simulink model "CrashAlgo_TestEnvironment_MotorradJan"  (R2019a)
settings: Solver=FixedStepAuto  StartTime=0.0  StopTime=data.timeVectorAcc(end)  FixedStep=0.01  RelTol=1e-3
undefined symbols (not defined in the file or in its folder): data, timeVector
libraries: simulink x1
settings Model: Creator=snj7rt  LastModifiedBy=snj7rt
settings DataIOCC: ReturnWorkspaceOutputs=off
settings DebuggingCC: ArithmeticOperatorsInVariantConditions=warning
settings SFSimCC: SimUseLocalCustomCode=off
settings RTWCC: RTWUseLocalCustomCode=off
settings CodeAppCC: StateflowObjectComments=on

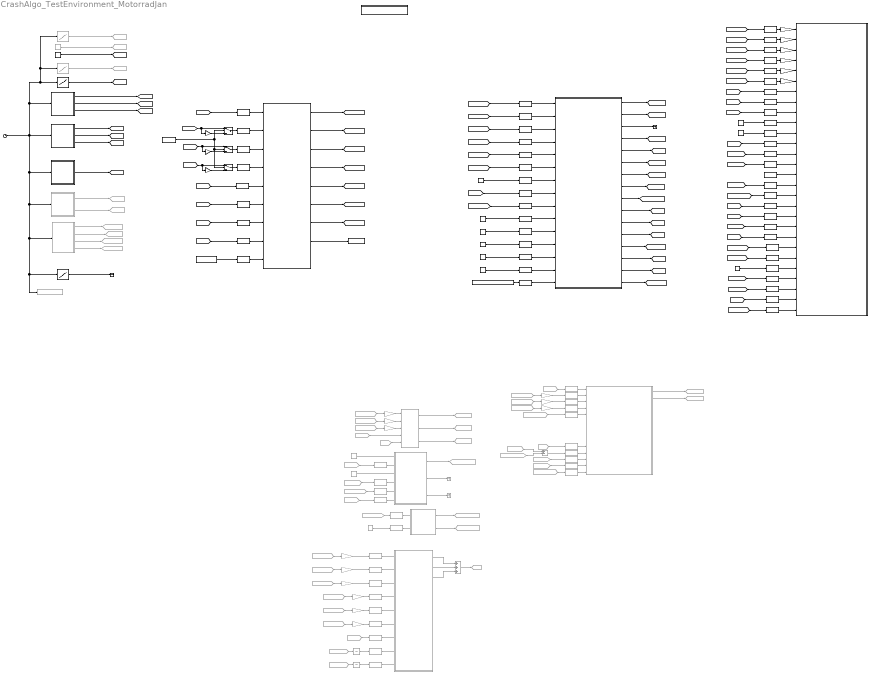
== system CrashAlgo_TestEnvironment_MotorradJan ==
  note: TestSetup for kalman extension regarding longitudinal acceleration compensation
  Acc_X1 : Lookup_n-D  Commented=on  NumberOfTableDimensions=1  BreakpointsForDimension1=timeVector(1:length([ones(floor(0.3*length(timeVector)),1);zeros(floor(0.7*length(timeVector)),1)]))  BreakpointsForDimension3=[5, 7]  Table=[20*ones(floor(0.3*length(timeVector)),1);zeros(floor(0.7*length(timeVector)),1)]  InternalRulePriority=Speed  RndMeth=Simplest  InputSameDT=on
  Accelerometer : Subsystem
  Add : Sum  Commented=on  Inputs=+-
  Add1 : Sum  Commented=on  Inputs=+++
  Barometer : Subsystem
  Chart1 : Stateflow chart  Commented=on  BlockKeywords=__PRM__SERIALIZED__DATA__:Stateflow Chart,Stateflow Diagram  TreatAsAtomicUnit=on
  Clock : Clock
  Constant : Constant  Value=data.osType
  Constant{1,3,8,11..12} (5 alike) : Constant  Value=0
  Constant10 : Constant  Value=data.InitRotMatFromLogFile
  Constant13 : Constant  Value=data.longAccCompForEulerEstFlagFromWorkspace
  Constant2 : Constant  Commented=on  Value=20
  Constant4 : Constant
  Constant46 : Constant  Commented=on  Value=10
  Constant47 : Constant  Commented=on  Value=0.1
  Constant5 : Constant  Value=2
  Constant6 : Constant  Value=5
  Constant7 : Constant  Value=7
  Constant9 : Constant  Commented=on  Value=2
  Data Type Conversion{,41,51..53,55..57,59..70,73,75} (22 alike) : DataTypeConversion  Commented=on  OutDataTypeStr=single
  Data Type Conversion{1..20,22..26,42..43,58} (28 alike) : DataTypeConversion
  Data Type Conversion{21,27..40,44..50,54,76} (24 alike) : DataTypeConversion  RndMeth=Zero
  Data Type Conversion71 : DataTypeConversion  Commented=on  OutDataTypeStr=int16
  Data Type Conversion72 : DataTypeConversion  Commented=on  OutDataTypeStr=int16
  Data Type Conversion74 : DataTypeConversion  Commented=on  OutDataTypeStr=int16
  Double-Click Button to set current folder : Subsystem
      settings: OpenFcn=cd(fileparts(get_param(gcs,'filename')));
      mask Display: disp('\bf\fontsize{16}Double-Click to set current folder      ','texmode','on')
  DuAcc : Subsystem  Commented=on
  FilterButterworth : Subsystem  Commented=on
  From{6,14,31,71} (4 alike) : From  Commented=on  GotoTag=StepTime
  From15 : From  Commented=on  GotoTag=accBfFiltX_g
  From18 : From  Commented=on  GotoTag=accBfFiltY_g
  From19 : From  Commented=on  GotoTag=accBfFiltZ_g
  From20 : From  Commented=on  GotoTag=accBf_X_mg
  From21 : From  Commented=on  GotoTag=accBf_Y_mg
  From22 : From  Commented=on  GotoTag=accBf_Z_mg
  From23 : From  Commented=on  GotoTag=accBfFiltX_g
  From30 : From  Commented=on  GotoTag=calibFlag
  From32 : From  Commented=on  GotoTag=reinitializeEulerEstimation
  From33 : From  Commented=on  GotoTag=SecondCalibrationDelayed
  From34 : From  Commented=on  GotoTag=gyrBf_X_mdegs
  From35 : From  Commented=on  GotoTag=gyrBf_Y_mdegs
  From36 : From  Commented=on  GotoTag=gyrBf_Z_mdegs
  From37 : From  Commented=on  GotoTag=gyrBf_X_mdegs
  From38 : From  Commented=on  GotoTag=eulerPitchComp_deg
  From39 : From  Commented=on  GotoTag=accBf_X_mg
  From40 : From  Commented=on  GotoTag=accBf_Y_mg
  From41 : From  Commented=on  GotoTag=accBf_Z_mg
  From42 : From  Commented=on  GotoTag=varSum
  From43 : From  Commented=on  GotoTag=varSum
  From44 : From  Commented=on  GotoTag=gyrBf_Y_mdegs
  From45 : From  Commented=on  GotoTag=gyrBf_Z_mdegs
  From47 : From  Commented=on  GotoTag=calibFlag
  From5 : From  Commented=on  GotoTag=Du_Speed
  From7 : From  Commented=on  GotoTag=longAccSpeedBased_g
  From95 : From  Commented=on  GotoTag=eulerRollComp_deg
  Gain{,1..5} (6 alike) : Gain  Gain=1/1000
  Gain{9..20} (12 alike) : Gain  Commented=on  Gain=1/1000
  Gain6 : Gain  Gain=-1
  Gain7 : Gain  Gain=-1
  Gain8 : Gain  Gain=-1
  Goto153 : Goto  Commented=on  GotoTag=longAccSpeedBased_g
  Goto16 : Goto  Commented=on  GotoTag=Du_Cadence
  Goto19 : Goto  Commented=on  GotoTag=Du_Speed
  Goto20 : Goto  Commented=on  GotoTag=initMountingAngleDeg
  Goto21 : Goto  Commented=on  GotoTag=accBfFiltX_g
  Goto22 : Goto  Commented=on  GotoTag=initMountingSetup
  Goto24 : Goto  Commented=on  GotoTag=DuAccX_mg
  Goto25 : Goto  Commented=on  GotoTag=DuAccZ_mg
  Goto26 : Goto  Commented=on  GotoTag=cobiHubConnection
  Goto27 : Goto  Commented=on  GotoTag=hubSetup
  Goto28 : Goto  Commented=on  GotoTag=accBfFiltY_g
  Goto29 : Goto  Commented=on  GotoTag=accBfFiltZ_g
  Goto3 : Goto  Commented=on  GotoTag=Du_Speed
  Goto30 : Goto  Commented=on  GotoTag=SecondCalibrationDelayed
  Goto31 : Goto  Commented=on  GotoTag=eulerRollComp_deg
  Goto32 : Goto  Commented=on  GotoTag=eulerPitchComp_deg
  Goto38 : Goto  Commented=on  GotoTag=varSum
  Goto57 : Goto  Commented=on  GotoTag=reinitializeEulerEstimation
  Gyroscope : Subsystem
  MATLAB Function : MATLAB Function  Commented=on  TreatAsAtomicUnit=on
  MATLAB Function2 : MATLAB Function  Commented=on  TreatAsAtomicUnit=on
  Model : ModelReference  ModelNameDialog=CalibrationMotorbike.slx  SimulationMode=Normal  ModelReferenceVersion=1.1438
  Model2 : ModelReference  ModelNameDialog=CRCL.slx  SimulationMode=Normal  ModelReferenceVersion=1.1949
  Model3 : ModelReference  ModelNameDialog=CrashAlgoSchnee_v2_analysis.slx  SimulationMode=Normal  ModelReferenceVersion=1.56
  SampleTime1 : Constant  Value=0.01
  Switch : Switch  Threshold=2
  Switch1 : Switch  Threshold=2
  Switch2 : Switch  Threshold=2
  Terminator : Terminator
  Terminator1 : Terminator
  Terminator2 : Terminator  Commented=on
  Terminator3 : Terminator  Commented=on
  To Workspace : ToWorkspace  VariableName=estRotMat  SampleTime=-1
  To Workspace2 : ToWorkspace  Commented=on  VariableName=simTimeVector  SampleTime=-1
      settings: Save2DSignal=2-D array (concatenate along first dimension)
  Unit Delay4 : UnitDelay  Commented=on  SampleTime=-1  HasFrameUpgradeWarning=on
  Unit Delay5 : UnitDelay  Commented=on  SampleTime=-1  HasFrameUpgradeWarning=on
  cadence : Lookup_n-D  Commented=on  NumberOfTableDimensions=1  BreakpointsForDimension1=data.timeVectorAcc  BreakpointsForDimension3=[5, 7]  Table=data.cadence_rpm  InternalRulePriority=Speed  RndMeth=Simplest  InputSameDT=on
  cobiSignals : Subsystem  Commented=on
  detectedCrashClass : Lookup_n-D  NumberOfTableDimensions=1  BreakpointsForDimension1=data.timeVectorAcc  BreakpointsForDimension3=[5, 7]  Table=data.crashClass  InternalRulePriority=Speed  RndMeth=Simplest  InputSameDT=on
  risingEdgeTrigger_RET : Stateflow chart  Commented=on  TreatAsAtomicUnit=on
  speed : Lookup_n-D  NumberOfTableDimensions=1  BreakpointsForDimension1=data.timeVectorAcc  BreakpointsForDimension3=[5, 7]  Table=data.speed_kmh  InternalRulePriority=Speed  RndMeth=Simplest  InputSameDT=on
  wires:
  Accelerometer/1(accSfX [mg]) -> [accSfX_mg]  "accSfXEnv_mg"
  Accelerometer/2(accSfY [mg]) -> [accSfY_mg]  "accSfYEnv_mg"
  Accelerometer/3(accSfZ [mg]) -> [accSfZ_mg]  "accSfZEnv_mg"
  Clock/1 -> cadence/1, Acc_X1/1, speed/1, Accelerometer/1(input_Time), Gyroscope/1(input_Time), DuAcc/1(input_Time), To Workspace2/1, detectedCrashClass/1, cobiSignals/1(In1), Barometer/1(input_Time)
  SampleTime1/1 -> [StepTime]
  Gyroscope/2(gyrSfY [mdeg/s]) -> [gyrSfY_mdegs]  "BMI_GYRO_Y"
  Gyroscope/1(gyrSfX [mdeg/s]) -> [gyrSfX_mdegs]  "BMI_GYRO_X"
  Gyroscope/3(gyrSfZ [mdeg/s]) -> [gyrSfZ_mdegs]  "BMI_GYRO_Z"
  Barometer/1(BME_pressure) -> [BMP_pressure]  "BME_pressure"
  Data Type Conversion14/1 -> Model3/15
  Data Type Conversion3/1 -> Gain1/1
  Data Type Conversion16/1 -> Model3/17
  Data Type Conversion9/1 -> Model3/8
  [eulerPitch_deg] -> Data Type Conversion42/1
  Data Type Conversion31/1 -> Model2/5
  [standFire] -> Data Type Conversion17/1
  Constant12/1 -> Data Type Conversion24/1
  [gyrBf_Y_mdegs] -> Data Type Conversion6/1
  Data Type Conversion19/1 -> Model3/20
  Data Type Conversion36/1 -> Model2/10
  Data Type Conversion29/1 -> Model2/3
  Data Type Conversion8/1 -> Model3/7
  Model2/6 -> [TO_curAngleDeg]
  Data Type Conversion5/1 -> Gain3/1
  Data Type Conversion42/1 -> Model3/9
  [gyrBf_X_mdegs] -> Data Type Conversion5/1
  [secondCalibDelayed] -> Data Type Conversion23/1
  [gyrBf_Z_mdegs] -> Data Type Conversion7/1
  [HD_collisionHitFire] -> Data Type Conversion15/1
  Constant5/1 -> Data Type Conversion36/1
  Data Type Conversion11/1 -> Model3/12
  Data Type Conversion28/1 -> Model2/2
  [calibFlag] -> Data Type Conversion22/1
  Data Type Conversion7/1 -> Gain5/1
  [HD_groundHitFire] -> Data Type Conversion13/1
  Model2/5 -> [TO_fire]
  [crashConfidenceLevel] -> Data Type Conversion26/1
  [Du_Speed] -> Data Type Conversion34/1
  [crashFire] -> Data Type Conversion19/1
  [StepTime] -> Data Type Conversion8/1
  Data Type Conversion32/1 -> Model2/6
  Model2/7 -> [HD_groundHitFire]
  Constant7/1 -> Data Type Conversion43/1
  Data Type Conversion43/1 -> Model3/10
  Data Type Conversion20/1 -> Model3/21
  Data Type Conversion15/1 -> Model3/16
  Constant6/1 -> Data Type Conversion10/1
  Data Type Conversion34/1 -> Model2/8
  Data Type Conversion27/1 -> Model2/1
  Data Type Conversion22/1 -> Model3/22
  Data Type Conversion23/1 -> Model3/23
  [RD_fire] -> Data Type Conversion18/1
  Data Type Conversion30/1 -> Model2/4
  Constant11/1 -> Data Type Conversion33/1
  Data Type Conversion17/1 -> Model3/18
  Data Type Conversion10/1 -> Model3/11
  Data Type Conversion6/1 -> Gain4/1
  [TO_curAngleDeg] -> Data Type Conversion12/1
  Data Type Conversion24/1 -> Model3/24
  Data Type Conversion25/1 -> Model3/25
  [HD_collisionHitCurVarSum] -> Data Type Conversion16/1
  [TO_fire] -> Data Type Conversion11/1
  [accBf_Z_mg] -> Data Type Conversion4/1
  Data Type Conversion2/1 -> Gain/1
  Data Type Conversion18/1 -> Model3/19
  [accBf_X_mg] -> Data Type Conversion2/1
  Model2/4 -> [crashConfidenceLevel]
  Model2/1 -> [crashFire]  "CrashFire"
  Data Type Conversion13/1 -> Model3/14
  Data Type Conversion35/1 -> Model2/9
  [eulerRoll_deg] -> Data Type Conversion9/1
  Data Type Conversion4/1 -> Gain2/1
  [accBf_Y_mg] -> Data Type Conversion3/1
  Data Type Conversion26/1 -> Model3/26
  [calibFlag] -> Data Type Conversion35/1
  [HD_hitDirection] -> Data Type Conversion20/1
  Data Type Conversion33/1 -> Model2/7
  Data Type Conversion12/1 -> Model3/13
  [Du_Speed] -> Data Type Conversion1/1
  Data Type Conversion1/1 -> Model3/27
  [BMP_pressure] -> Data Type Conversion45/1
  Data Type Conversion45/1 -> Model/1
  Data Type Conversion46/1 -> Model/2
  Data Type Conversion47/1 -> Model/3
  Data Type Conversion21/1 -> Model/4
  Data Type Conversion44/1 -> Model/5
  Data Type Conversion48/1 -> Model/6
  Data Type Conversion49/1 -> Model/7
  Data Type Conversion50/1 -> Model/8
  Constant2/1 -> Goto3/1
  Model/1 -> [accBf_X_mg]
  Model/2 -> [accBf_Y_mg]
  Model/3 -> [accBf_Z_mg]
  Model/4 -> [gyrBf_X_mdegs]
  Model/5 -> [gyrBf_Y_mdegs]
  Model/6 -> [gyrBf_Z_mdegs]
  Model/7 -> [calibFlag]
  speed/1 -> [Du_Speed]
  [Du_Speed] -> Data Type Conversion50/1
  Acc_X1/1 -> Goto19/1
  Data Type Conversion40/1 -> Model2/14
  Constant3/1 -> Data Type Conversion40/1
  [accBf_X_mg] -> Data Type Conversion27/1
  [accBf_Y_mg] -> Data Type Conversion28/1
  [accBf_Z_mg] -> Data Type Conversion29/1
  [gyrBf_X_mdegs] -> Data Type Conversion30/1
  [gyrBf_Y_mdegs] -> Data Type Conversion31/1
  [gyrBf_Z_mdegs] -> Data Type Conversion32/1
  [SmartphoneDropOutFire] -> Data Type Conversion58/1
  Data Type Conversion58/1 -> Model3/28
  Model2/2 -> [crashScenario]
  [crashScenario] -> Data Type Conversion25/1
  detectedCrashClass/1 -> Terminator/1  "savedCrashClass"
  cobiSignals/1(cobiHubConnection) -> Goto26/1
  cobiSignals/2(cobiHubSetup) -> Goto27/1
  cobiSignals/3(cobiMountingAngle) -> Goto20/1  "InitMountingAngle"
  cobiSignals/4(cobiMountingSetup) -> Goto22/1
  DuAcc/1(DuAccX  [mg]) -> Goto24/1
  DuAcc/2(DuAccZ [mg]) -> Goto25/1
  Model2/3 -> Terminator1/1
  Model2/16 -> [SmartphoneDropOutFire]
  cadence/1 -> Goto16/1
  Gain/1 -> Model3/1
  Gain1/1 -> Model3/2
  Gain2/1 -> Model3/3
  Gain3/1 -> Model3/4
  Gain4/1 -> Model3/5
  Gain5/1 -> Model3/6
  Constant1/1 -> Data Type Conversion37/1
  Data Type Conversion37/1 -> Model2/11
  Constant4/1 -> Data Type Conversion38/1
  Data Type Conversion38/1 -> Model2/12
  Constant8/1 -> Data Type Conversion39/1
  Data Type Conversion39/1 -> Model2/13
  Data Type Conversion54/1 -> Model/9
  Constant10/1 -> Data Type Conversion54/1
  Model/8 -> To Workspace/1
  Model2/8 -> [HD_collisionHitFire]
  Model2/9 -> [HD_collisionHitCurVarSum]
  Model2/10 -> [standFire]
  Model2/11 -> [RD_fire]
  Model2/12 -> [HD_hitDirection]
  Model2/13 -> [secondCalibDelayed]
  Model2/14 -> [eulerPitch_deg]
  Model2/15 -> [eulerRoll_deg]
  [accSfX_mg] -> Gain6/1, Switch/1
  [accSfY_mg] -> Gain7/1, Switch1/1
  [accSfZ_mg] -> Gain8/1, Switch2/1
  [gyrSfZ_mdegs] -> Data Type Conversion49/1
  [gyrSfY_mdegs] -> Data Type Conversion48/1
  Switch1/1 -> Data Type Conversion47/1
  Switch2/1 -> Data Type Conversion21/1
  [gyrSfX_mdegs] -> Data Type Conversion44/1
  Switch/1 -> Data Type Conversion46/1
  Constant/1 -> Switch2/2, Switch1/2, Switch/2
  Gain6/1 -> Switch/3
  Gain7/1 -> Switch1/3
  Gain8/1 -> Switch2/3
  Constant46/1 -> Chart1/1(LAE_minSpeed_kmh)
  Chart1/1(LAE_longAcc_g) -> Goto153/1  "LAE_longAcc_g"
  Constant47/1 -> Chart1/3(LAE_minSpeedDelta_kmh)
  From5/1 -> Data Type Conversion/1
  MATLAB Function/1(pitch_deg) -> Goto31/1  "pitchKalmanAccComp_deg"
  From6/1 -> Data Type Conversion41/1
  FilterButterworth/3(Z_filt) -> Goto29/1  "accBfFiltZ"
  FilterButterworth/1(X_filt) -> Goto21/1  "accBfFiltX"
  FilterButterworth/2(Y_filt) -> Goto28/1  "accBfFiltY"
  From22/1 -> Gain11/1
  From21/1 -> Gain9/1
  From20/1 -> Gain10/1
  Gain10/1 -> FilterButterworth/1(X)
  Gain9/1 -> FilterButterworth/2(Y)
  Gain11/1 -> FilterButterworth/3(Z)
  From14/1 -> FilterButterworth/4(SampleTime)
  From18/1 -> Data Type Conversion59/1
  From19/1 -> Data Type Conversion60/1
  risingEdgeTrigger_RET/1(RET_output) -> Goto57/1  "reinitEulerEstimation"
  From47/1 -> Data Type Conversion71/1
  risingEdgeTrigger_RET/2(RET_OutDelayed) -> Goto30/1  "secCalibDone Delayed"
  Constant9/1 -> Data Type Conversion72/1  "delayTime"
  From33/1 -> Data Type Conversion61/1
  From32/1 -> Data Type Conversion55/1
  From35/1 -> Gain13/1
  From34/1 -> Gain12/1
  From36/1 -> Gain14/1
  Gain12/1 -> Data Type Conversion51/1
  Gain13/1 -> Data Type Conversion52/1
  Gain14/1 -> Data Type Conversion53/1
  Add/1 -> Data Type Conversion57/1  "accBfXKalmanIn_g"
  From7/1 -> Add/2
  From15/1 -> Add/1
  Gain20/1 -> Data Type Conversion66/1
  Gain17/1 -> Data Type Conversion64/1
  Unit Delay5/1 -> Data Type Conversion70/1
  Gain16/1 -> Data Type Conversion63/1
  Gain18/1 -> Data Type Conversion65/1
  From38/1 -> Unit Delay5/1
  Add1/1 -> Goto38/1  "accVarSum"
  Unit Delay4/1 -> Data Type Conversion69/1
  Gain15/1 -> Data Type Conversion62/1
  From71/1 -> Data Type Conversion68/1
  Gain19/1 -> Data Type Conversion67/1
  MATLAB Function2/1(varAccX) -> Add1/1  "varAccX"
  MATLAB Function2/2(varAccY) -> Add1/2  "varAccY"
  From95/1 -> Unit Delay4/1
  From42/1 -> FilterButterworth/5("accVarSum ")
  From43/1 -> Data Type Conversion56/1
  MATLAB Function2/3(varAccZ) -> Add1/3  "varAccZ"
  From44/1 -> Gain16/1
  From45/1 -> Gain17/1
  From37/1 -> Gain15/1
  From39/1 -> Gain18/1
  From41/1 -> Gain19/1
  From40/1 -> Gain20/1
  MATLAB Function/2(roll_deg) -> Goto32/1  "rollKalmanAccComp_deg"
  Data Type Conversion41/1 -> MATLAB Function/1(timeStep_s)
  Data Type Conversion51/1 -> MATLAB Function/2(gyrX_degs)
  Data Type Conversion52/1 -> MATLAB Function/3(gyrY_degs)
  Data Type Conversion53/1 -> MATLAB Function/4(gyrZ_degs)
  Data Type Conversion55/1 -> MATLAB Function/5(reinitializeFlag)
  Data Type Conversion56/1 -> MATLAB Function/10(varSum)
  Data Type Conversion57/1 -> MATLAB Function/11(accBfFiltX_g)
  Data Type Conversion59/1 -> MATLAB Function/12(accBfFiltY_g)
  Data Type Conversion60/1 -> MATLAB Function/13(accBfFiltZ_g)
  Data Type Conversion61/1 -> MATLAB Function/14(secondCalibrationIsDone)
  Data Type Conversion62/1 -> MATLAB Function2/1(gyrX)
  Data Type Conversion63/1 -> MATLAB Function2/2(gyrY)
  Data Type Conversion64/1 -> MATLAB Function2/3(gyrZ)
  Data Type Conversion65/1 -> MATLAB Function2/4(accX)
  Data Type Conversion66/1 -> MATLAB Function2/5(accY)
  Data Type Conversion67/1 -> MATLAB Function2/6(accZ)
  Data Type Conversion68/1 -> MATLAB Function2/7(stepTime_s)
  Data Type Conversion69/1 -> MATLAB Function2/8(roll_deg)
  Data Type Conversion70/1 -> MATLAB Function2/9(pitch_deg)
  Data Type Conversion71/1 -> risingEdgeTrigger_RET/1(RET_curValue)
  Data Type Conversion72/1 -> risingEdgeTrigger_RET/2(RET_Latchtime)
  From23/1 -> Data Type Conversion73/1
  Data Type Conversion73/1 -> Chart1/4(LAE_curAccBfXFilt_g)
  Chart1/2(LAE_longAccTmp_g) -> Terminator2/1  "LAE_longAccTmp_g"
  From30/1 -> Data Type Conversion74/1
  Data Type Conversion74/1 -> Chart1/5(LAE_curCalibState)
  Data Type Conversion/1 -> Chart1/2(LAE_curSpeed_kmh)
  From31/1 -> Data Type Conversion75/1
  Data Type Conversion75/1 -> Chart1/6(LAE_timeStep_s)
  Chart1/3(LAE_timer_s) -> Terminator3/1  "LAE_timer_s"
  Constant13/1 -> Data Type Conversion76/1
  Data Type Conversion76/1 -> Model2/15

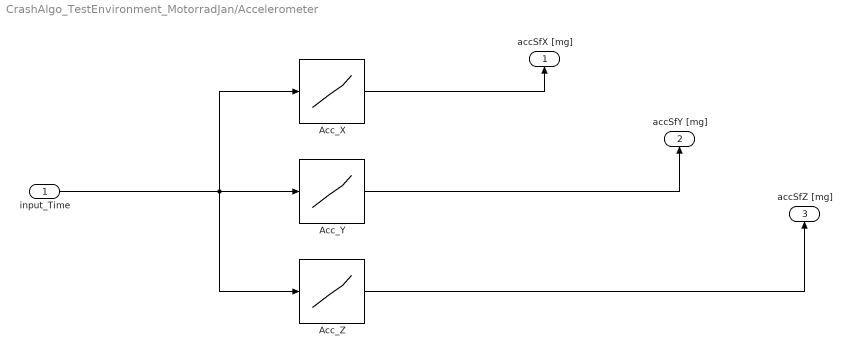
== system CrashAlgo_TestEnvironment_MotorradJan/Accelerometer ==
  input_Time : Inport
  Acc_X : Lookup_n-D  NumberOfTableDimensions=1  BreakpointsForDimension1=data.timeVectorAcc  BreakpointsForDimension3=[5, 7]  Table=data.AccSfX_mg  InternalRulePriority=Speed  RndMeth=Simplest  InputSameDT=on
  Acc_Y : Lookup_n-D  NumberOfTableDimensions=1  BreakpointsForDimension1=data.timeVectorAcc  BreakpointsForDimension3=[5, 7]  Table=data.AccSfY_mg  InternalRulePriority=Speed  RndMeth=Simplest  InputSameDT=on
  Acc_Z : Lookup_n-D  NumberOfTableDimensions=1  BreakpointsForDimension1=data.timeVectorAcc  BreakpointsForDimension3=[5, 7]  Table=data.AccSfZ_mg  InternalRulePriority=Speed  RndMeth=Simplest  InputSameDT=on
  accSfX [mg] : Outport
  accSfY [mg] : Outport  Port=2
  accSfZ [mg] : Outport  Port=3
  wires:
  input_Time/1 -> Acc_Z/1, Acc_Y/1, Acc_X/1
  Acc_X/1 -> accSfX [mg]/1
  Acc_Z/1 -> accSfZ [mg]/1
  Acc_Y/1 -> accSfY [mg]/1

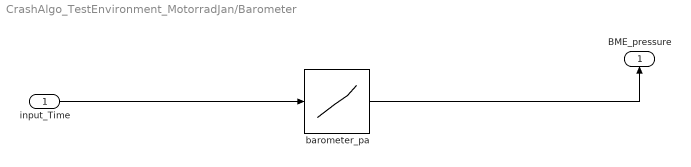
== system CrashAlgo_TestEnvironment_MotorradJan/Barometer ==
  input_Time : Inport
  barometer_pa : Lookup_n-D  NumberOfTableDimensions=1  BreakpointsForDimension1=data.timeVectorAcc  BreakpointsForDimension3=[5, 7]  Table=data.barometer_pa  InternalRulePriority=Speed  RndMeth=Simplest  InputSameDT=on
  BME_pressure : Outport
  wires:
  input_Time/1 -> barometer_pa/1
  barometer_pa/1 -> BME_pressure/1

== system CrashAlgo_TestEnvironment_MotorradJan/Double-Click Button to set current folder ==

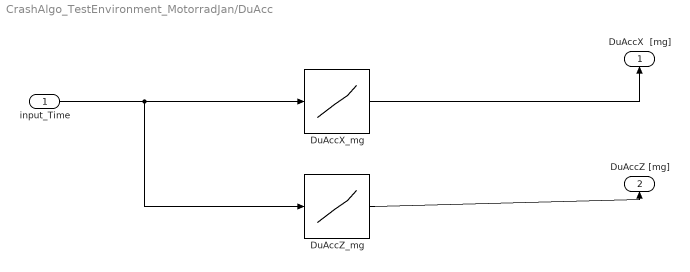
== system CrashAlgo_TestEnvironment_MotorradJan/DuAcc ==
  input_Time : Inport
  DuAccX_mg : Lookup_n-D  NumberOfTableDimensions=1  BreakpointsForDimension1=data.timeVectorAcc  BreakpointsForDimension3=[5, 7]  Table=data.DuAccX_mg  InternalRulePriority=Speed  RndMeth=Simplest  InputSameDT=on
  DuAccZ_mg : Lookup_n-D  NumberOfTableDimensions=1  BreakpointsForDimension1=data.timeVectorAcc  BreakpointsForDimension3=[5, 7]  Table=data.DuAccZ_mg  InternalRulePriority=Speed  RndMeth=Simplest  InputSameDT=on
  DuAccX  [mg] : Outport
  DuAccZ [mg] : Outport  Port=2
  wires:
  DuAccX_mg/1 -> DuAccX  [mg]/1
  input_Time/1 -> DuAccZ_mg/1, DuAccX_mg/1
  DuAccZ_mg/1 -> DuAccZ [mg]/1

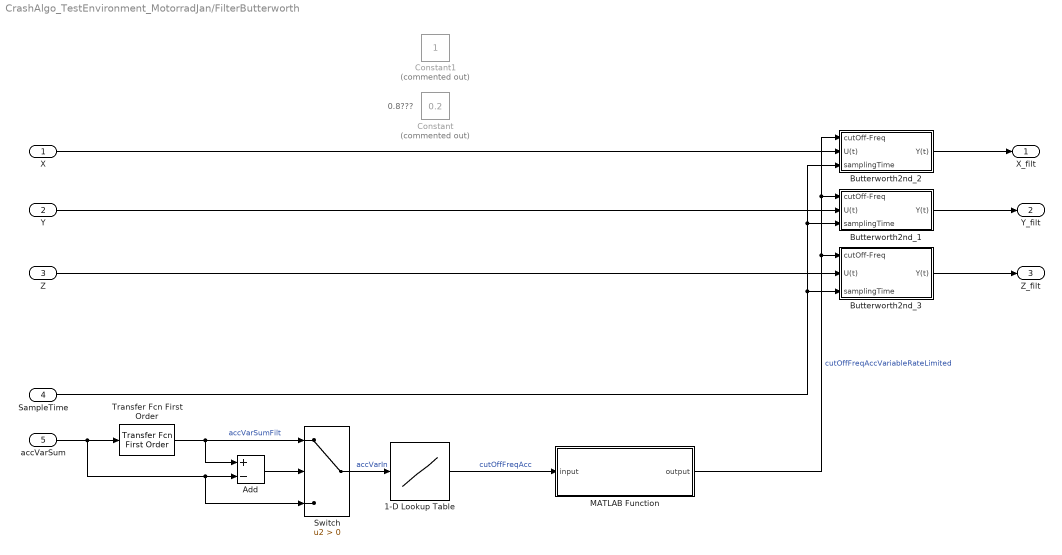
== system CrashAlgo_TestEnvironment_MotorradJan/FilterButterworth ==
  note: 0.8???
  X : Inport
  Y : Inport  Port=2
  Z : Inport  Port=3
  SampleTime : Inport  Port=4
  "accVarSum " : Inport  Port=5
  1-D Lookup Table : Lookup_n-D  NumberOfTableDimensions=1  BreakpointsForDimension1=[0 0.0005 0.005 0.01 0.1 50]  Table=[10 10 1 0.5 0.2 0.2]  InternalRulePriority=Speed  RndMeth=Simplest  InputSameDT=on
  Add : Sum  Inputs=+-
  Butterworth2nd_1 : Subsystem
  Butterworth2nd_2 : Subsystem
  Butterworth2nd_3 : Subsystem
  Constant : Constant  Commented=on  Value=0.2  OutDataTypeStr=single
  Constant1 : Constant  Commented=on
  MATLAB Function : MATLAB Function  TreatAsAtomicUnit=on
  Switch : Switch  Criteria=u2 > Threshold
  Transfer Fcn First Order : simulink/Discrete/Transfer Fcn First Order  PoleZ=0.92  ICPrevOutput=0.0  DoSatur=off
      settings: SourceProductName=Simulink
  X_filt : Outport
  Y_filt : Outport  Port=2
  Z_filt : Outport  Port=3
  wires:
  Butterworth2nd_2/1(Y(t)) -> X_filt/1
  Butterworth2nd_1/1(Y(t)) -> Y_filt/1
  Butterworth2nd_3/1(Y(t)) -> Z_filt/1
  Z/1 -> Butterworth2nd_3/2(U(t))
  Y/1 -> Butterworth2nd_1/2(U(t))
  X/1 -> Butterworth2nd_2/2(U(t))
  "accVarSum "/1 -> Switch/3, Add/2, Transfer Fcn First Order/1
  Add/1 -> Switch/2
  Transfer Fcn First Order/1 -> Add/1, Switch/1  "accVarSumFilt"
  Switch/1 -> 1-D Lookup Table/1  "accVarIn"
  1-D Lookup Table/1 -> MATLAB Function/1(input)  "cutOffFreqAcc"
  MATLAB Function/1(output) -> Butterworth2nd_2/1(cutOff-Freq), Butterworth2nd_1/1(cutOff-Freq), Butterworth2nd_3/1(cutOff-Freq)  "cutOffFreqAccVariableRateLimited"
  SampleTime/1 -> Butterworth2nd_1/3(samplingTime), Butterworth2nd_2/3(samplingTime), Butterworth2nd_3/3(samplingTime)

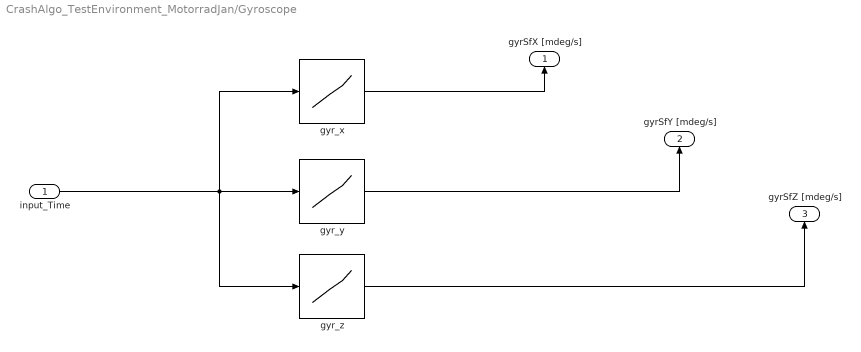
== system CrashAlgo_TestEnvironment_MotorradJan/Gyroscope ==
  input_Time : Inport
  gyr_x : Lookup_n-D  NumberOfTableDimensions=1  BreakpointsForDimension1=data.timeVectorGyr  BreakpointsForDimension3=[5, 7]  Table=data.GyrSfX_mdegs  InternalRulePriority=Speed  RndMeth=Simplest  InputSameDT=on
  gyr_y : Lookup_n-D  NumberOfTableDimensions=1  BreakpointsForDimension1=data.timeVectorGyr  BreakpointsForDimension3=[5, 7]  Table=data.GyrSfY_mdegs  InternalRulePriority=Speed  RndMeth=Simplest  InputSameDT=on
  gyr_z : Lookup_n-D  NumberOfTableDimensions=1  BreakpointsForDimension1=data.timeVectorGyr  BreakpointsForDimension3=[5, 7]  Table=data.GyrSfZ_mdegs  InternalRulePriority=Speed  RndMeth=Simplest  InputSameDT=on
  gyrSfX [mdeg/s] : Outport
  gyrSfY [mdeg/s] : Outport  Port=2
  gyrSfZ [mdeg/s] : Outport  Port=3
  wires:
  input_Time/1 -> gyr_y/1, gyr_z/1, gyr_x/1
  gyr_x/1 -> gyrSfX [mdeg/s]/1
  gyr_y/1 -> gyrSfY [mdeg/s]/1
  gyr_z/1 -> gyrSfZ [mdeg/s]/1

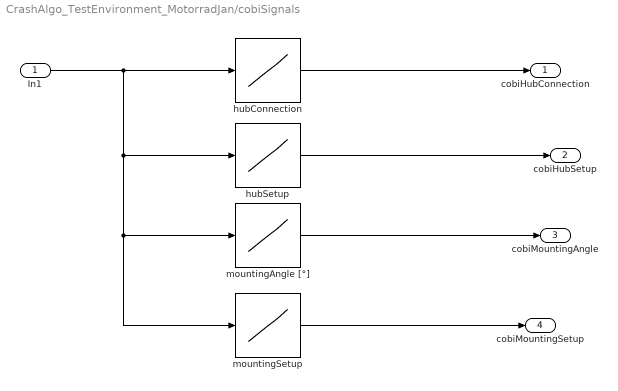
== system CrashAlgo_TestEnvironment_MotorradJan/cobiSignals ==
  In1 : Inport
  hubConnection : Lookup_n-D  NumberOfTableDimensions=1  BreakpointsForDimension1=data.timeVectorAcc  BreakpointsForDimension3=[5, 7]  Table=data.hubConnection  InternalRulePriority=Speed  RndMeth=Simplest  InputSameDT=on
  hubSetup : Lookup_n-D  NumberOfTableDimensions=1  BreakpointsForDimension1=data.timeVectorAcc  BreakpointsForDimension3=[5, 7]  Table=data.cobiHubSetup  InternalRulePriority=Speed  RndMeth=Simplest  InputSameDT=on
  mountingAngle [°] : Lookup_n-D  NumberOfTableDimensions=1  BreakpointsForDimension1=data.timeVectorAcc  BreakpointsForDimension3=[5, 7]  Table=data.mountingAngle  InternalRulePriority=Speed  RndMeth=Simplest  InputSameDT=on
  mountingSetup : Lookup_n-D  NumberOfTableDimensions=1  BreakpointsForDimension1=data.timeVectorAcc  BreakpointsForDimension3=[5, 7]  Table=data.mountingSetup  InternalRulePriority=Speed  RndMeth=Simplest  InputSameDT=on
  cobiHubConnection : Outport
  cobiHubSetup : Outport  Port=2
  cobiMountingAngle : Outport  Port=3
  cobiMountingSetup : Outport  Port=4
  wires:
  hubSetup/1 -> cobiHubSetup/1
  mountingSetup/1 -> cobiMountingSetup/1
  mountingAngle [°]/1 -> cobiMountingAngle/1
  In1/1 -> hubSetup/1, mountingAngle [°]/1, mountingSetup/1, hubConnection/1
  hubConnection/1 -> cobiHubConnection/1

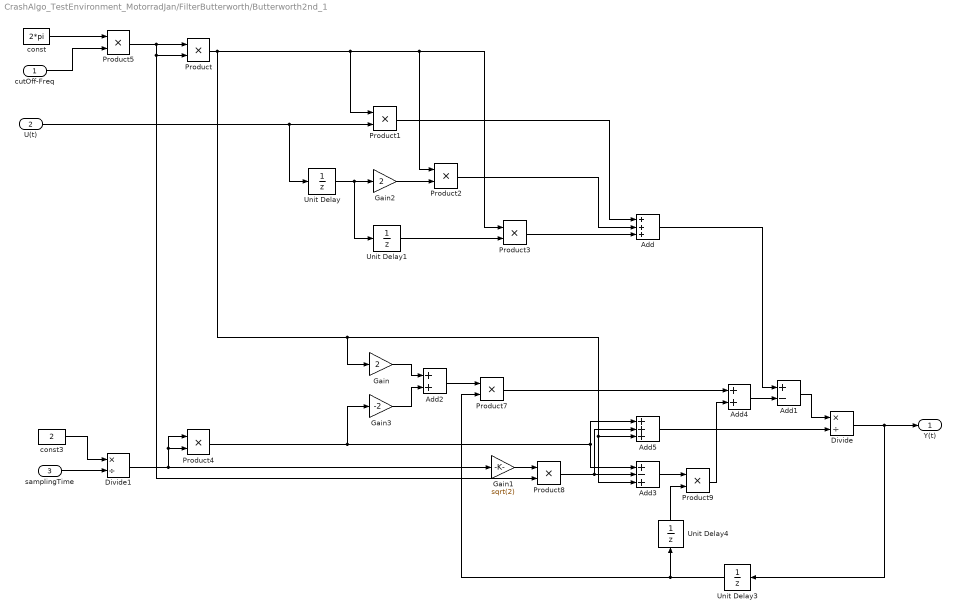
== system CrashAlgo_TestEnvironment_MotorradJan/FilterButterworth/Butterworth2nd_1 ==
  cutOff-Freq : Inport
  U(t) : Inport  Port=2
  samplingTime : Inport  Port=3
  Add : Sum  Inputs=+++
  Add1 : Sum  Inputs=+-
  Add2 : Sum
  Add3 : Sum  Inputs=+-+
  Add4 : Sum
  Add5 : Sum  Inputs=+++
  Divide : Product  Inputs=*/
  Divide1 : Product  Inputs=*/
  Gain : Gain  Gain=2
  Gain1 : Gain  Gain=sqrt(2)
  Gain2 : Gain  Gain=2
  Gain3 : Gain  Gain=-2
  Product{,1..5,7..9} (9 alike) : Product  RndMeth=Zero
  Unit Delay{,1,3..4} (4 alike) : UnitDelay  SampleTime=-1  HasFrameUpgradeWarning=on
  const : Constant  Value=2*pi  OutDataTypeStr=single
  const3 : Constant  Value=2  OutDataTypeStr=single
  Y(t) : Outport
  wires:
  U(t)/1 -> Product1/2, Unit Delay/1
  Product/1 -> Product1/1, Product3/1, Product2/1, Gain/1, Add3/3, Add5/3
  Unit Delay/1 -> Unit Delay1/1, Gain2/1
  Unit Delay1/1 -> Product3/2
  Product1/1 -> Add/1
  Product2/1 -> Add/2
  Product3/1 -> Add/3
  Add/1 -> Add1/1
  Divide/1 -> Unit Delay3/1, Y(t)/1
  Product4/1 -> Add3/1, Add5/1, Gain3/1
  Gain/1 -> Add2/1
  Unit Delay3/1 -> Product7/2, Unit Delay4/1
  Add2/1 -> Product7/1
  Gain1/1 -> Product8/1
  Product8/1 -> Add3/2, Add5/2
  Unit Delay4/1 -> Product9/2
  Add3/1 -> Product9/1
  Product9/1 -> Add4/2
  Product7/1 -> Add4/1
  Add4/1 -> Add1/2
  Add1/1 -> Divide/1
  Add5/1 -> Divide/2
  Gain2/1 -> Product2/2
  Gain3/1 -> Add2/2
  Product5/1 -> Product/1, Product/2, Product8/2
  const/1 -> Product5/1
  cutOff-Freq/1 -> Product5/2
  const3/1 -> Divide1/1
  samplingTime/1 -> Divide1/2
  Divide1/1 -> Gain1/1, Product4/2, Product4/1

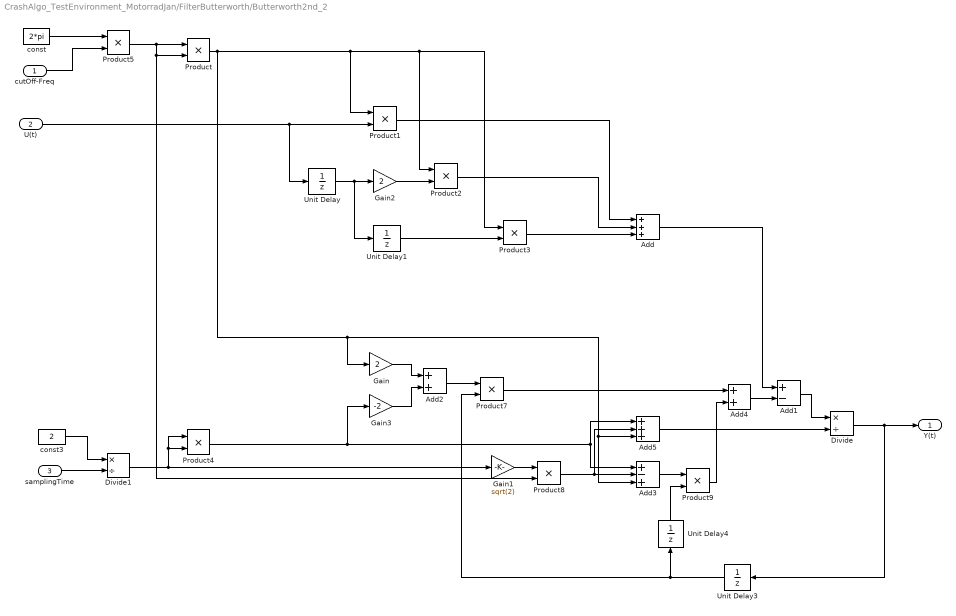
== system CrashAlgo_TestEnvironment_MotorradJan/FilterButterworth/Butterworth2nd_2 ==
  cutOff-Freq : Inport
  U(t) : Inport  Port=2
  samplingTime : Inport  Port=3
  Add : Sum  Inputs=+++
  Add1 : Sum  Inputs=+-
  Add2 : Sum
  Add3 : Sum  Inputs=+-+
  Add4 : Sum
  Add5 : Sum  Inputs=+++
  Divide : Product  Inputs=*/
  Divide1 : Product  Inputs=*/
  Gain : Gain  Gain=2
  Gain1 : Gain  Gain=sqrt(2)
  Gain2 : Gain  Gain=2
  Gain3 : Gain  Gain=-2
  Product{,1..5,7..9} (9 alike) : Product  RndMeth=Zero
  Unit Delay{,1,3..4} (4 alike) : UnitDelay  SampleTime=-1  HasFrameUpgradeWarning=on
  const : Constant  Value=2*pi  OutDataTypeStr=single
  const3 : Constant  Value=2  OutDataTypeStr=single
  Y(t) : Outport
  wires:
  Divide1/1 -> Product4/1, Product4/2, Gain1/1
  samplingTime/1 -> Divide1/2
  const3/1 -> Divide1/1
  cutOff-Freq/1 -> Product5/2
  const/1 -> Product5/1
  Product5/1 -> Product8/2, Product/2, Product/1
  Gain3/1 -> Add2/2
  Gain2/1 -> Product2/2
  Add5/1 -> Divide/2
  Add1/1 -> Divide/1
  Add4/1 -> Add1/2
  Product7/1 -> Add4/1
  Product9/1 -> Add4/2
  Add3/1 -> Product9/1
  Unit Delay4/1 -> Product9/2
  Product8/1 -> Add5/2, Add3/2
  Gain1/1 -> Product8/1
  Add2/1 -> Product7/1
  Unit Delay3/1 -> Unit Delay4/1, Product7/2
  Gain/1 -> Add2/1
  Product4/1 -> Gain3/1, Add5/1, Add3/1
  Divide/1 -> Y(t)/1, Unit Delay3/1
  Add/1 -> Add1/1
  Product3/1 -> Add/3
  Product2/1 -> Add/2
  Product1/1 -> Add/1
  Unit Delay1/1 -> Product3/2
  Unit Delay/1 -> Gain2/1, Unit Delay1/1
  Product/1 -> Add5/3, Add3/3, Gain/1, Product2/1, Product3/1, Product1/1
  U(t)/1 -> Unit Delay/1, Product1/2

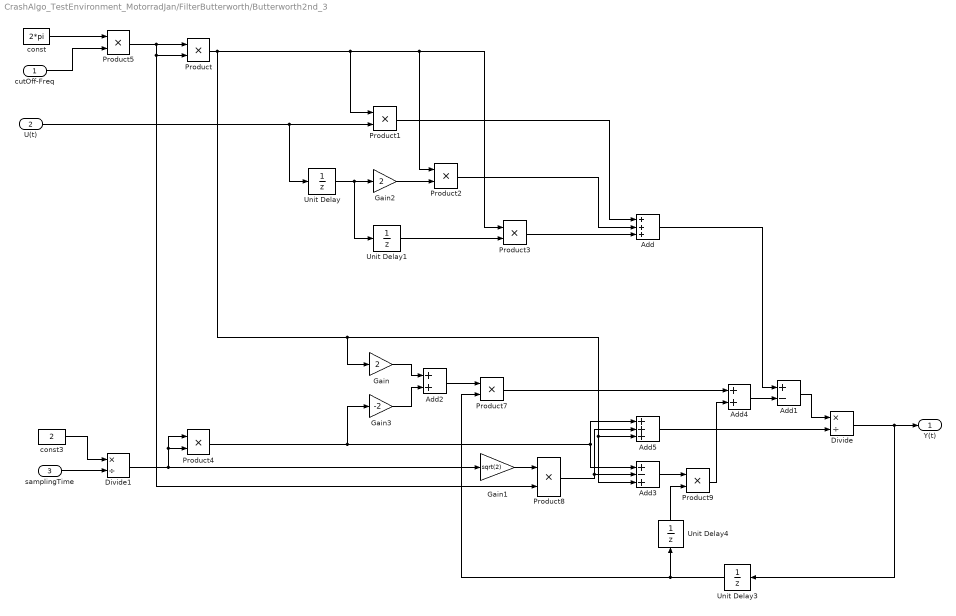
== system CrashAlgo_TestEnvironment_MotorradJan/FilterButterworth/Butterworth2nd_3 ==
  cutOff-Freq : Inport
  U(t) : Inport  Port=2
  samplingTime : Inport  Port=3
  Add : Sum  Inputs=+++
  Add1 : Sum  Inputs=+-
  Add2 : Sum
  Add3 : Sum  Inputs=+-+
  Add4 : Sum
  Add5 : Sum  Inputs=+++
  Divide : Product  Inputs=*/
  Divide1 : Product  Inputs=*/
  Gain : Gain  Gain=2
  Gain1 : Gain  Gain=sqrt(2)
  Gain2 : Gain  Gain=2
  Gain3 : Gain  Gain=-2
  Product{,1..5,7..9} (9 alike) : Product  RndMeth=Zero
  Unit Delay{,1,3..4} (4 alike) : UnitDelay  SampleTime=-1  HasFrameUpgradeWarning=on
  const : Constant  Value=2*pi  OutDataTypeStr=single
  const3 : Constant  Value=2  OutDataTypeStr=single
  Y(t) : Outport
  wires:
  Divide1/1 -> Product4/1, Product4/2, Gain1/1
  samplingTime/1 -> Divide1/2
  const3/1 -> Divide1/1
  cutOff-Freq/1 -> Product5/2
  const/1 -> Product5/1
  Product5/1 -> Product8/2, Product/2, Product/1
  Gain3/1 -> Add2/2
  Gain2/1 -> Product2/2
  Add5/1 -> Divide/2
  Add1/1 -> Divide/1
  Add4/1 -> Add1/2
  Product7/1 -> Add4/1
  Product9/1 -> Add4/2
  Add3/1 -> Product9/1
  Unit Delay4/1 -> Product9/2
  Product8/1 -> Add5/2, Add3/2
  Gain1/1 -> Product8/1
  Add2/1 -> Product7/1
  Unit Delay3/1 -> Unit Delay4/1, Product7/2
  Gain/1 -> Add2/1
  Product4/1 -> Gain3/1, Add5/1, Add3/1
  Add/1 -> Add1/1
  Product3/1 -> Add/3
  Product2/1 -> Add/2
  Product1/1 -> Add/1
  Unit Delay1/1 -> Product3/2
  Unit Delay/1 -> Gain2/1, Unit Delay1/1
  Product/1 -> Add5/3, Add3/3, Gain/1, Product2/1, Product3/1, Product1/1
  U(t)/1 -> Unit Delay/1, Product1/2
  Divide/1 -> Unit Delay3/1, Y(t)/1

== matlab function CrashAlgo_TestEnvironment_MotorradJan/MATLAB Function2 ==
  data: gyrX input; gyrY input; gyrZ input; accX input; accY input; accZ input; varAccX output; varAccY output; varAccZ output; varGyrX output; varGyrY output; varGyrZ output; impulseX output; impulseY output; impulseZ output; stepTime_s input; extremaAccValY output; roll_deg input; pitch_deg input; impulseShortTermX output; impulseShortTermY output
function [varAccX, varAccY, varAccZ, ...
    varGyrX, varGyrY, varGyrZ, ...
    impulseX, impulseY, impulseZ, ...
    extremaAccValY, ...
    impulseShortTermX, impulseShortTermY] = ...
    varPastNumSamples(gyrX, gyrY, gyrZ, ...
    accX, accY, accZ, stepTime_s, roll_deg, pitch_deg)

persistent ringBufAccX ringBufAccY ringBufAccZ i ringBufXgComp ringBufYgComp ...
    ringBufZgComp NumSamplesLongtermIntern NumSamplesShortTermIntern ...
    ringBufGyrX ringBufGyrY ringBufGyrZ
        
%% declaration only during first run!
gCompensation = 1;

if isempty(i)  
        NumSamplesLongtermIntern = int16(7);
        NumSamplesShortTermIntern = int16(5);
        
%% for crash feature evaluation --> different buffer sizes...
%         ringBufX = single(zeros(NumSamplesLongtermIntern,1));
%         ringBufY = single(zeros(NumSamplesLongtermIntern,1));
%         ringBufZ = single(zeros(NumSamplesLongtermIntern,1));
%         ringBufYgComp = single(zeros(NumSamplesLongtermIntern,1));
%         ringBufXgComp = single(zeros(NumSamplesLongtermIntern,1));
%         ringBufZgComp = single(zeros(NumSamplesLongtermIntern,1));
%         ringBufmaxImpulseZ = single(zeros(NumlatchedImpulseZ,1));
%%
        ringBufAccX = single(zeros(7,1));   % variable from NumSamplesLongtermIntern
        ringBufAccY = single(zeros(7,1));   % variable from NumSamplesLongtermIntern
        ringBufAccZ = single(zeros(7,1));   % variable from NumSamplesLongtermIntern
        ringBufXgComp = single(zeros(7,1)); % variable from NumSamplesLongtermIntern
        ringBufYgComp = single(zeros(7,1)); % variable from NumSamplesLongtermIntern
        ringBufZgComp = single(zeros(7,1)); % variable from NumSamplesLongtermIntern
        ringBufGyrX = single(zeros(7,1));   % variable from NumSamplesLongtermIntern
        ringBufGyrY = single(zeros(7,1));   % variable from NumSamplesLongtermIntern
        ringBufGyrZ = single(zeros(7,1));   % variable from NumSamplesLongtermIntern
        
        i = int16(1); 
end

ringBufAccX(i) = accX;
ringBufAccY(i) = accY;
ringBufAccZ(i) = accZ;

ringBufGyrX(i) = gyrX;
ringBufGyrY(i) = gyrY;
ringBufGyrZ(i) = gyrZ;

ringBufXgComp(i) = accX + sind(pitch_deg);
ringBufYgComp(i) = accY - sind(roll_deg);
ringBufZgComp(i) = accZ - cosd(pitch_deg);



varAccX = single(var(ringBufAccX, 0));
varAccY = single(var(ringBufAccY, 0));
varAccZ = single(var(ringBufAccZ, 0));


varGyrX = single(var(ringBufGyrX, 0));
varGyrY = single(var(ringBufGyrY, 0));
varGyrZ = single(var(ringBufGyrZ, 0));



%% for crash feature evaluation --> different buffer sizes...
% indicesMutedLatchedImpulseZ = b-4:b;
% 
% for a=1:length(indicesMutedLatchedImpulseZ)
%     if indicesMutedLatchedImpulseZ(a) <= 0
%         indicesMutedLatchedImpulseZ(a) = indicesMutedLatchedImpulseZ(a)+ NumlatchedImpulseZ;
%     end
% end


%indicesShortTerm = i-(NumSamplesShortTermIntern-1):i;

% for a=1:length(indicesShortTerm)
%     if indicesShortTerm(a) <= 0
%         indicesShortTerm(a) = indicesShortTerm(a)+ NumSamplesLongtermIntern;
%     end
% end

%%

indicesShortTerm = int16(zeros(5,1));   % variable from NumSamplesShortTermIntern
indicesShortTerm(1) = i-4;
indicesShortTerm(2) = i-3;
indicesShortTerm(3) = i-2;
indicesShortTerm(4) = i-1;
indicesShortTerm(5) = i;

for a=1:5
    if indicesShortTerm(a) <= 0
        indicesShortTerm(a) = indicesShortTerm(a)+ NumSamplesLongtermIntern;
    end
end


if  gCompensation == 1
    impulseX = sum(ringBufXgComp.*stepTime_s);
    impulseY = sum(ringBufYgComp.*stepTime_s);
    impulseZ = sum(ringBufZgComp.*stepTime_s);
    impulseShortTermX = sum(ringBufXgComp(indicesShortTerm).*stepTime_s);
    impulseShortTermY = sum(ringBufYgComp(indicesShortTerm).*stepTime_s);
    %impulseShortTermZ = sum(ringBufAccZ(indicesShortTerm).*stepTime_s);
else
    impulseX = sum(ringBufAccX.*stepTime_s);
    impulseY = sum(ringBufAccY.*stepTime_s);
    impulseZ = sum(ringBufAccZ.*stepTime_s);
    impulseShortTermX = sum(ringBufAccX(indicesShortTerm).*stepTime_s);
    impulseShortTermY = sum(ringBufAccY(indicesShortTerm).*stepTime_s);
    %impulseShortTermZ = sum(ringBufAccZ(indicesShortTerm).*stepTime_s);
end

[extremaAccValY, extremaIndY] = max(abs(ringBufAccY));
if sign(ringBufAccY(extremaIndY)) == 1
    %extremaAccValY = extremaAccValY;
else
    extremaAccValY = extremaAccValY * -1;
end

i = i + 1;
if i > NumSamplesLongtermIntern
    i = int16(1);
end

end

== matlab function CrashAlgo_TestEnvironment_MotorradJan/MATLAB Function ==
  data: pitch_deg output; timeStep_s input; roll_deg output; gyrX_degs input; gyrY_degs input; gyrZ_degs input; innovationPitch output; innovationRoll output; pitchGyroPredict output; rollGyroPredict output; pitchAcc output; rollAcc output; gyrBiasX output; gyrBiasY output; reinitializeFlag input; SD_fire input; HD_GroundHit input; HD_CollisionHit input; TO_fire input; varSum input; accBfFiltX_g input; accBfFiltY_g input; accBfFiltZ_g input; u1 output; secondCalibrationIsDone input; u2 output
function [pitch_deg, roll_deg, innovationPitch, innovationRoll, ...
    pitchGyroPredict, rollGyroPredict, pitchAcc, rollAcc, ...
    gyrBiasX, gyrBiasY, u1, u2] ...
    = kalman1(timeStep_s, ...
    gyrX_degs, gyrY_degs, gyrZ_degs, reinitializeFlag, ...
    SD_fire, HD_GroundHit, HD_CollisionHit, TO_fire, varSum, ...
    accBfFiltX_g, accBfFiltY_g, accBfFiltZ_g, secondCalibrationIsDone)

%accBf_g = [accBfX_g; accBfY_g; accBfZ_g];
accBf_g = [accBfFiltX_g; accBfFiltY_g; accBfFiltZ_g];
accBf_g = accBf_g/norm(accBf_g);

%check Data: if Accelerometer is all zero, Kalman Filter returns NaN
if ~any(accBf_g) 
    accBf_g = single([0.05; 0.05; 1]);
end

dt = timeStep_s;


persistent x P A B H R Q I betaGyroBias gyrBiasMeasuredX gyrBiasMeasuredY ...
    lastAccPitch lastAccRoll

%% declaration only during first run!

if isempty(x)
    noise_accel = single(1e-1);  %1e-1
    noise_gyro = single(8e-7);   %5e-7
    x = single([0; 0]);      % Initial State (pitch and roll angle)
    P = single([1000, 0;...
        0, 1000]);       % Initial Uncertainty
    A = single([1, 0;...
        0, 1]);        % Transition Matrix
    B = single([dt, 0; ...
        0, dt]);         %control matrix -> gyro input evaluation
    H = single([1, 0; ...
        0, 1]);       % Measurement function
    R = single([noise_accel, 0;...
        0, noise_accel]);             % measurement noise covariance
    Q = single([noise_gyro, 0;...
        0, noise_gyro]); % Process Noise Covariance
    I = single(eye(2));             % Identity matrix
    gyrBiasMeasuredX = single(0);
    gyrBiasMeasuredY = single(0);
    betaGyroBias = single(1e-7);  
    lastAccPitch = single(0);
    lastAccRoll = single(0);
end

gyrBf_degs = [gyrX_degs-gyrBiasMeasuredX; gyrY_degs-gyrBiasMeasuredY; gyrZ_degs];

if reinitializeFlag == 1
    noise_accel = single(5e-3);
    R_intern = single([noise_accel, 0;...
        0, noise_accel]);   
elseif SD_fire && (HD_GroundHit == 1 || HD_CollisionHit >= 2 || TO_fire == 1)
    noise_accel = single(5e-4);
    R_intern = single([noise_accel, 0;...
        0, noise_accel]);  
elseif varSum < 0.0002
    noise_accel = single(5e-3);
    R_intern = single([noise_accel, 0;...
        0, noise_accel]);  
else
    R_intern = R;
end

if varSum > 0.0001 || sum(abs(x)) > 20
    betaGyroBiasIntern = betaGyroBias;
else
    betaGyroBiasIntern = single(5e-6);
end

Q_intern = Q;
% if  badEulerEstimationCounter >=  5000
%     noise_gyro = single(1e-4);   %5e-7
%      Q_intern = single([noise_gyro, 0;...
%         0, noise_gyro]); % Process Noise Covariance
%     noise_accel = single(5e-5);
%     R_intern = single([noise_accel, 0;...
%         0, noise_accel]);   
%     accBf_g = [accBfFiltX_g; accBfFiltY_g; accBfFiltZ_g];
% else 
%     Q_intern = Q;
% end
    
% gyro input data    
% u = [gyrY_degs-gyrBiasMeasuredY;gyrX_degs-gyrBiasMeasuredX];
% u = [(gyrY_degs-gyrBiasMeasuredY)*cosd(x(2))-gyrZ_degs*sind(x(2)); ...
%    gyrX_degs-gyrBiasMeasuredX];
% u = [(gyrY_degs-gyrBiasMeasuredY)*cosd(x(2))-gyrZ_degs*sind(x(2)); ...
%     (gyrX_degs-gyrBiasMeasuredX)*cosd(x(1))-gyrZ_degs*sind(x(1))];



%rotate Data into navigation frame see: https://de.wikipedia.org/wiki/Eulersche_Winkel
gyrNf_degs = [cosd(x(1)) 0 sind(x(1)); ...
    0 1 0; ...
    -sind(x(1)) 0 cosd(x(1))] * ...
    [1 0 0; ...
    0 cosd(x(2)) -sind(x(2));
    0 sind(x(2)) cosd(x(2))] * gyrBf_degs;

u=[gyrNf_degs(2); gyrNf_degs(1)];
u1 = u(1);
u2 = u(2);

% Prediction    
x_predict = A * x + B * u;                  % Prädizierter Zustand aus Bisherigem und System
P = A * P * A' + Q_intern;             % Prädizieren der Kovarianz


% quatAcc = [0 accBf_g'];
% quatAcc = quatAcc./norm(quatAcc);
% euler = quatern2euler(quatAcc)*180/pi;
% rollAcc = euler(1);
% pitchAcc = euler(2);

%rollAcc = atand(accBf_g(2)/accBf_g(3));
rollAcc = atand(accBf_g(2)/sqrt(accBf_g(3)^2+accBf_g(1)^2));
if accBf_g(3) < - 0.3 && abs(accBf_g(1)) < 0.6 && accBf_g(2) > 0 && abs(lastAccPitch) < 100
    rollAcc = -rollAcc+180;  
elseif accBf_g(3) < - 0.3 && abs(accBf_g(1)) < 0.6 && accBf_g(2) < 0 && abs(lastAccPitch) < 100
    rollAcc = -rollAcc-180; 
elseif accBf_g(1) < -0.1 && abs(accBf_g(1)) > abs(accBf_g(3))
    %rollAcc = -1*rollAcc;  
end

pitchAcc = -1*atand(accBf_g(1)/sqrt(accBf_g(3)^2+accBf_g(2)^2));
if accBf_g(3) < -0.3 && abs(accBf_g(2)) < 0.6 && accBf_g(1) > 0 && abs(lastAccRoll) < 100
    pitchAcc = -pitchAcc-180;
elseif accBf_g(3) < -0.3 && abs(accBf_g(2)) < 0.6 && accBf_g(1) < 0 && abs(lastAccRoll) < 100
    pitchAcc = -pitchAcc+180;
elseif accBf_g(3) < 0 && accBf_g(1) < 0
    %pitchAcc = -1*pitchAcc;
end


% Correction

Z = [pitchAcc; rollAcc];
y = Z - (H * x_predict);              % Innovation aus Messwertdifferenz
%y = Z - x_predict;     
S = (H * P * H' + R_intern);           % Innovationskovarianz
K = P * H' * inv(S);          % Filter-Matrix (Kalman-Gain)

x = x_predict + (K * y);              % aktualisieren des Systemzustands
P = (I - (K * H)) * P;          % aktualisieren der Kovarianz


%Bias Estimation
if secondCalibrationIsDone == 1 && sqrt(x_predict(1)^2+x_predict(2)^2) <= 25 && ...
        sqrt((x(1) - pitchAcc)^2 + (x(2) - rollAcc)^2) <= 30
    gyrBiasMeasuredY = (1-betaGyroBiasIntern) * gyrBiasMeasuredY + betaGyroBiasIntern*(x(1) - pitchAcc)/dt;
    gyrBiasMeasuredX = (1-betaGyroBiasIntern)  * gyrBiasMeasuredX + betaGyroBiasIntern*(x(2) - rollAcc)/dt;
    %max gyro bias of bmi160 is declared as 3°/s -> saturate bias
    %estimation, in case of misfunction
    gyrBiasMeasuredX = saturateKalman(gyrBiasMeasuredX, 4);  
    gyrBiasMeasuredY = saturateKalman(gyrBiasMeasuredY, 4);
end

pitchGyroPredict = x_predict(1);
rollGyroPredict = x_predict(2);

innovationPitch = y(1);
innovationRoll = y(2);

%unwrap pitchAngle
if x(1) > 180 
    x(1) = x(1)-360;    
elseif x(1) < -180
    x(1) = x(1)+360;
elseif (x(1) > 165 && pitchAcc < -165) || (x(1) < -165 && pitchAcc > 165)
    x(1) = -x(1); 
end

%unwrap rollAngle
if x(2) > 180 
    x(2) = x(2)-360;   
elseif x(2) < -180 
    x(2) = x(2)+360;
elseif (x(2) > 165 && rollAcc < -165) || (x(2) < -165 && rollAcc > 165)
    x(2) = -x(2); 
end

pitch_deg = x(1);
roll_deg = x(2);

gyrBiasX = gyrBiasMeasuredX;
gyrBiasY = gyrBiasMeasuredY;

debugOut = single(0);

lastAccRoll = rollAcc;
lastAccPitch = pitchAcc;

end


function euler = quatern2euler(q)
%QUATERN2EULER Converts a quaternion orientation to ZYX Euler angles
%
%   q = quatern2euler(q)
%
%   Converts a quaternion orientation to ZYX Euler angles where phi is a
%   rotation around X, theta around Y and psi around Z.
%
%   For more information see:
%   http://www.x-io.co.uk/node/8#quaternions
%
%	Date          Author          Notes
%	27/09/2011    SOH Madgwick    Initial release
% R = zeros(3,3,1);
%     R(1,1,:) = 2.*q(:,1).^2-1+2.*q(:,2).^2;
%     R(2,1,:) = 2.*(q(:,2).*q(:,3)-q(:,1).*q(:,4));
%     R(3,1,:) = 2.*(q(:,2).*q(:,4)+q(:,1).*q(:,3));
%     R(3,2,:) = 2.*(q(:,3).*q(:,4)-q(:,1).*q(:,2));
%     R(3,3,:) = 2.*q(:,1).^2-1+2.*q(:,4).^2;
% 
%     phi = atan2(R(3,2,:), R(3,3,:) );
%     theta = -atan(R(3,1,:) ./ sqrt(1-R(3,1,:).^2) );
%     psi = atan2(R(2,1,:), R(1,1,:) );
% 
%     euler = [phi(1,:)' theta(1,:)' psi(1,:)'];
    
    R = zeros(3,3);
    R(1,1) = 2.*q(1).^2-1+2.*q(2).^2;
    R(2,1) = 2.*(q(2).*q(3)-q(1).*q(4));
    R(3,1) = 2.*(q(2).*q(4)+q(1).*q(3));
    R(3,2) = 2.*(q(3).*q(4)-q(1).*q(2));
    R(3,3) = 2.*q(1).^2-1+2.*q(4).^2;

    phi = atan2(R(3,2), R(3,3));
    theta = -atan(R(3,1) ./ sqrt(1-R(3,1).^2) );
    psi = atan2(R(2,1), R(1,1) );

    euler = [phi theta psi];
end

function output = saturateKalman(input, limit)
%output = single(0);
 if input > limit
     output = single(limit);
 elseif input < -1*limit
     output = single(-1*limit);
 else
     output = single(input);
 end

end

== stateflow chart CrashAlgo_TestEnvironment_MotorradJan/risingEdgeTrigger_RET ==
  state Init
    en:
    RET_lastValue = int16(0);
    RET_OutDelayed = int16(0);
  state Idle
  state waitState
    en:
    RET_output = int16(1);
  state End
    during:
    RET_lastValue = RET_curValue;
  (default) -> Init
  Init -> Idle
  End -> waitState : %reinitialize euler estimation
      | [RET_curValue == 2 && RET_lastValue == 1]
  Idle -> waitState [order 1] : [RET_lastValue == 0 && RET_curValue >= 1]
  Idle -> (junction 6) [order 2] : {
      | RET_output = int16(0);
      | }
  (junction 6) -> Idle : {
      | RET_lastValue = RET_curValue;
      | }
  waitState -> End : [after(RET_Latchtime,sec)]
      | {
      | RET_output = int16(0);
      | RET_OutDelayed = int16(1);
      | }
  data: RET_curValue input; RET_output output; RET_lastValue local; RET_OutDelayed output; RET_Latchtime input

== matlab function CrashAlgo_TestEnvironment_MotorradJan/FilterButterworth/MATLAB Function ==
  data: input input; output output
function output = variabelRateLimiter(input)

persistent lastOutput

if isempty(lastOutput)
   lastOutput = single(0); 
end

if input >= lastOutput || lastOutput <= 0.4 || 1/15*(lastOutput-input) <= 0.025
    output = input;
else
    if 1/5*(lastOutput-input) > 0.4
        output = lastOutput-1/5*(lastOutput-input);
    else
        output = lastOutput-1/15*(lastOutput-input);
    end
end

lastOutput = output;
end

== stateflow chart CrashAlgo_TestEnvironment_MotorradJan/Chart1 ==
  state EstimateLongitudinalAcceleration [parallel]
    settings: executionOrder=1
    state speedChange
      en:
      if LAE_timer_s < 2
      LAE_longAccTmp_g = (LAE_curSpeed_kmh-LAE_lastSpeed_kmh)/(3.6*9.81*LAE_timer_s);
      else
      LAE_longAccTmp_g = (LAE_curSpeed_kmh-LAE_lastSpeed_kmh)/(3.6*9.81);
      end
      LAE_lastSpeed_kmh = LAE_curSpeed_kmh;
      LAE_timerReset = int16(1);
      if LAE_longAccTmp_g > LAE_curAccBfXFilt_g && LAE_curAccBfXFilt_g > 0 && LAE_longAccTmp_g > 0
      LAE_longAcc_g = LAE_curAccBfXFilt_g;
      elseif LAE_longAccTmp_g < LAE_curAccBfXFilt_g && LAE_curAccBfXFilt_g < 0 && LAE_longAccTmp_g < 0
      LAE_longAcc_g = LAE_curAccBfXFilt_g;
      elseif sign(LAE_curAccBfXFilt_g) ~= sign(LAE_longAccTmp_g)
      LAE_longAcc_g = single(0);
      else
      LAE_longAcc_g = LAE_longAccTmp_g;
      end
      du:
      %if filtered accX signal is still changing
      if LAE_longAccTmp_g > LAE_curAccBfXFilt_g && LAE_curAccBfXFilt_g > 0 && LAE_longAccTmp_g > 0
      LAE_longAcc_g = LAE_curAccBfXFilt_g;
      elseif LAE_longAccTmp_g < LAE_curAccBfXFilt_g && LAE_curAccBfXFilt_g < 0 && LAE_longAccTmp_g < 0
      LAE_longAcc_g = LAE_curAccBfXFilt_g;
      elseif sign(LAE_curAccBfXFilt_g) ~= sign(LAE_longAccTmp_g)
      LAE_longAcc_g = single(0);
      else
      LAE_longAcc_g = LAE_longAccTmp_g;
      end
    state Idle
      du:
      LAE_lastSpeed_kmh = LAE_curSpeed_kmh;
    speedChange -> speedChange [commented out] : %accelerating
        | [LAE_curSpeed_kmh-LAE_lastSpeed_kmh > LAE_minSpeedDelta_kmh && ...
        |  LAE_lastSpeed_kmh >= LAE_minSpeed_kmh && ...
        | LAE_curCalibState == 1]
    speedChange -> speedChange [commented out] : %decelerating
        | [LAE_lastSpeed_kmh-LAE_curSpeed_kmh > LAE_minSpeedDelta_kmh && ...
        | (LAE_curSpeed_kmh >= LAE_minSpeed_kmh || ...
        |  LAE_lastSpeed_kmh >= LAE_minSpeed_kmh) && ...
        | LAE_curCalibState == 1]
    (default) -> Idle : {
        | LAE_lastSpeed_kmh = single(0);
        | LAE_longAcc_g = single(0);
        | LAE_longAccTmp_g = single(0);
        | }
    Idle -> speedChange [commented out] : %decelerating
        | [LAE_lastSpeed_kmh-LAE_curSpeed_kmh > LAE_minSpeedDelta_kmh && ...
        | (LAE_curSpeed_kmh >= LAE_minSpeed_kmh || ...
        |  LAE_lastSpeed_kmh >= LAE_minSpeed_kmh) && ...
        | LAE_curCalibState == 1]
    Idle -> speedChange [commented out] : %accelerating
        | [LAE_curSpeed_kmh-LAE_lastSpeed_kmh > LAE_minSpeedDelta_kmh && ...
        |  LAE_lastSpeed_kmh >= LAE_minSpeed_kmh && ...
        | LAE_curCalibState == 1]
    Idle -> speedChange : [abs(LAE_curSpeed_kmh-LAE_lastSpeed_kmh) > LAE_minSpeedDelta_kmh && ...
        |  (LAE_curSpeed_kmh >= LAE_minSpeed_kmh || ...
        |  LAE_lastSpeed_kmh >= LAE_minSpeed_kmh) && ...
        | LAE_curCalibState == 1]
    speedChange -> Idle [order 2] : [after(1.05,sec)] %GPS speed rate ~1Hz
        | {
        | LAE_longAcc_g = single(0);
        | LAE_longAccTmp_g = single(0);
        | }
    speedChange -> speedChange [order 1] : [abs(LAE_curSpeed_kmh-LAE_lastSpeed_kmh) > LAE_minSpeedDelta_kmh && ...
        |  (LAE_curSpeed_kmh >= LAE_minSpeed_kmh || ...
        |  LAE_lastSpeed_kmh >= LAE_minSpeed_kmh) && ...
        | LAE_curCalibState == 1]
  state SpeedUpdateTime [parallel]
    settings: executionOrder=2
    state Counter
      en:
      LAE_timer_s = single(0);
      LAE_timerReset = int16(0);
      du:
      LAE_timer_s = LAE_timer_s + LAE_timeStep_s;
    (default) -> Counter
    Counter -> Counter : [LAE_timerReset == 1]
  data: LAE_minSpeed_kmh input; LAE_curSpeed_kmh input; LAE_minSpeedDelta_kmh input; LAE_longAcc_g output; LAE_lastSpeed_kmh local; LAE_curAccBfXFilt_g input; LAE_longAccTmp_g output; LAE_curCalibState input; LAE_timeStep_s input; LAE_timerReset local; LAE_timer_s output
